simulink model "pid_pid_normal"  (Simulink 7.6)
settings: Solver=ode45  StartTime=0.0  StopTime=500  RelTol=1e-3
settings Model: Creator=Administrator  LastModifiedBy=Administrator

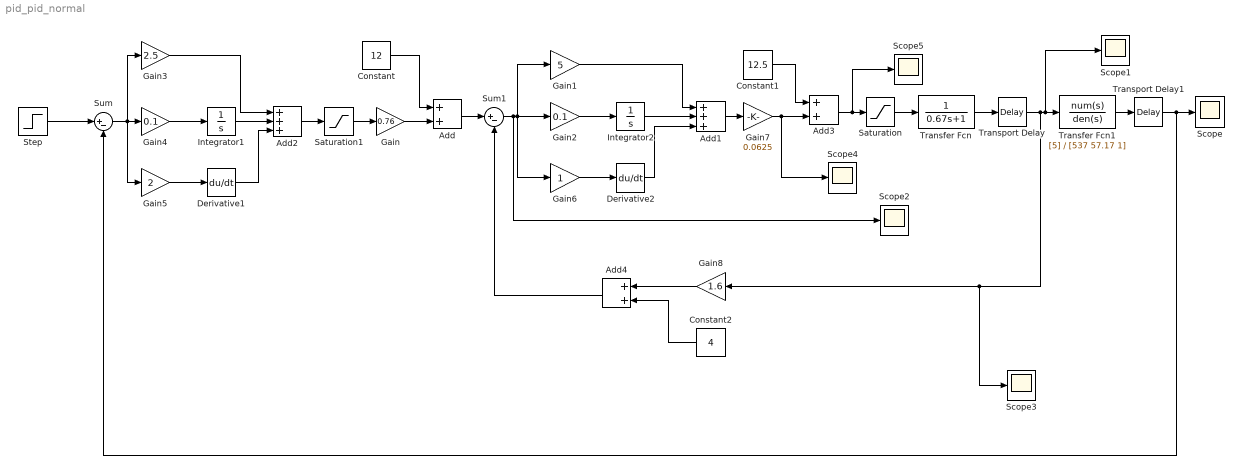
== system pid_pid_normal ==
  Add : Sum
  Add1 : Sum  Inputs=+++
  Add2 : Sum  Inputs=+++
  Add3 : Sum
  Add4 : Sum
  Constant : Constant  Value=12
  Constant1 : Constant  Value=12.5
  Constant2 : Constant  Value=4
  Derivative1 : Derivative
  Derivative2 : Derivative
  Gain : Gain  Gain=0.76
  Gain1 : Gain  Gain=5
  Gain2 : Gain  Gain=0.1
  Gain3 : Gain  Gain=2.5
  Gain4 : Gain  Gain=0.1
  Gain5 : Gain  Gain=2
  Gain6 : Gain
  Gain7 : Gain  Gain=0.0625
  Gain8 : Gain  Gain=1.6
  Integrator1 : Integrator
  Integrator2 : Integrator
  Saturation : Saturate  UpperLimit=10  LowerLimit=-10
  Saturation1 : Saturate  UpperLimit=50  LowerLimit=-50
  Scope{,1..5} (6 alike) : Scope
      Scope settings: TimeRange=500  YMin=48.78573  YMax=53.92107
      Scope2 settings: SaveName=ScopeData2
      Scope3 settings: SaveName=ScopeData3
      Scope4 settings: SaveName=ScopeData4
      Scope5 settings: SaveName=ScopeData5
  Step : Step  Time=0  After=50  SampleTime=0
  Sum : Sum  Inputs=|+-
  Sum1 : Sum  Inputs=|+-
  Transfer Fcn : TransferFcn  Denominator=[0.67 1]
  Transfer Fcn1 : TransferFcn  Numerator=[5]  Denominator=[537 57.17 1]
  Transport Delay : TransportDelay  DelayTime=0.058
  Transport Delay1 : TransportDelay  DelayTime=11.85
  wires:
  Gain4/1 -> Integrator1/1
  Integrator1/1 -> Add2/2
  Derivative1/1 -> Add2/3
  Gain3/1 -> Add2/1
  Gain5/1 -> Derivative1/1
  Add2/1 -> Saturation1/1
  Sum/1 -> Gain5/1, Gain4/1, Gain3/1
  Gain2/1 -> Integrator2/1
  Integrator2/1 -> Add1/2
  Derivative2/1 -> Add1/3
  Gain1/1 -> Add1/1
  Gain6/1 -> Derivative2/1
  Add1/1 -> Gain7/1
  Add/1 -> Sum1/1
  Gain/1 -> Add/2
  Constant/1 -> Add/1
  Sum1/1 -> Gain2/1, Gain6/1, Gain1/1, Scope2/1
  Gain7/1 -> Add3/2, Scope4/1
  Constant1/1 -> Add3/1
  Add3/1 -> Saturation/1, Scope5/1
  Transfer Fcn/1 -> Transport Delay/1
  Transport Delay/1 -> Transfer Fcn1/1, Scope1/1, Gain8/1, Scope3/1
  Transfer Fcn1/1 -> Transport Delay1/1
  Transport Delay1/1 -> Scope/1, Sum/2
  Saturation/1 -> Transfer Fcn/1
  Saturation1/1 -> Gain/1
  Step/1 -> Sum/1
  Constant2/1 -> Add4/2
  Gain8/1 -> Add4/1
  Add4/1 -> Sum1/2
